simulink model "Target_Control_System"  (R2021b)
settings: Solver=FixedStepDiscrete  StartTime=0.0  StopTime=5  RelTol=1e-3
PreLoadFcn:
  | RTWConfigurationCB('preloadfcn', bdroot);
PostLoadFcn:
  | load('configuration/data_struct.mat');
  | load('configuration/fluxMaps_propMotor.mat');
  | load('configuration/parameterInit_PROP.mat');
  | load('configuration/parameterInit_PUMP.mat');
  | load('configuration/parameterInit_PITCH.mat');
  | load('configuration/parameterInit_TILT.mat');
  | %load('configuration/base_workspace_signal_definition.mat');
  | %load('resolvedatastores_to_baseworkspace_for_faster_simulation.mat');
model workspace (MAT data in the model file):
  SIMULATION_OPTIONS : Simulink.Parameter (value not decoded)
  TARGET_CODE_GEN : Simulink.Parameter (value not decoded)
  TCS_SAMPLE_FREQ_HZ : Simulink.Parameter (value not decoded)
symbols that are objects in the model workspace (value not decoded): TARGET_CODE_GEN, TCS_SAMPLE_FREQ_HZ
undefined symbols (not defined in the file): A_DQ_REF_LPF_INIT__PITCH, A_DQ_REF_LPF_INIT__PROP, A_DQ_REF_LPF_INIT__PUMP, A_DQ_REF_LPF_INIT__TILT, A_OBSERVER_CONFIDENCE_INIT__PITCH, A_OBSERVER_CONFIDENCE_INIT__PROP, A_OBSERVER_CONFIDENCE_INIT__PUMP, A_OBSERVER_CONFIDENCE_INIT__TILT, ACTUATOR_MAX_ANGLE_TRIP__PITCH, ACTUATOR_MIN_ANGLE_TRIP__PITCH, ACTUATOR_POS_SENSOR_INV_DIRECTION__PITCH, ACTUATOR_POS_SENSOR_INV_DIRECTION__TILT, ACTUATOR_POS_SENSOR_OFFSET__PITCH, ACTUATOR_POS_SENSOR_OFFSET__TILT, ADC_scaler1_baseaddr_TILT, ADC_SCALER_FLOAT_TO_FIXPOINT_EXPANSION, ANGLE_ELEC_FROM_SENSOR_OFFSET_INIT__PITCH, ANGLE_ELEC_FROM_SENSOR_OFFSET_INIT__PROP, ANGLE_ELEC_FROM_SENSOR_OFFSET_INIT__PUMP, ANGLE_ELEC_FROM_SENSOR_OFFSET_INIT__TILT, AUTO_CLEAR_FAULTS_ENABLED__PITCH, AUTO_CLEAR_FAULTS_ENABLED__PROP, AUTO_CLEAR_FAULTS_ENABLED__PUMP, AUTO_CLEAR_FAULTS_ENABLED__TILT, AUTO_CLEAR_FAULTS_WAIT_TICKS__PITCH, AUTO_CLEAR_FAULTS_WAIT_TICKS__PROP, AUTO_CLEAR_FAULTS_WAIT_TICKS__PUMP, AUTO_CLEAR_FAULTS_WAIT_TICKS__TILT, AUTO_I_ZERO_IDLE_TICKS__PITCH, AUTO_I_ZERO_IDLE_TICKS__PROP, AUTO_I_ZERO_IDLE_TICKS__PUMP, AUTO_I_ZERO_IDLE_TICKS__TILT, AUTO_I_ZERO_OFFSET_IDC_THRESHOLD__PITCH, AUTO_I_ZERO_OFFSET_IDC_THRESHOLD__PROP, AUTO_I_ZERO_OFFSET_IDC_THRESHOLD__PUMP, AUTO_I_ZERO_OFFSET_IDC_THRESHOLD__TILT, AUTO_I_ZERO_OFFSET_IPH_THRESHOLD__PITCH, AUTO_I_ZERO_OFFSET_IPH_THRESHOLD__PROP, AUTO_I_ZERO_OFFSET_IPH_THRESHOLD__PUMP, AUTO_I_ZERO_OFFSET_IPH_THRESHOLD__TILT, AUTO_SENSORLESS_SWITCHOVER_DISABLE_OMEGA, AUTO_SENSORLESS_SWITCHOVER_ENABLE_OMEGA, AUTO_SENSORLESS_SWITCHOVER_MIN_CONFIDENCE, AUXILIARY_PROTECTION_UNIT_BASEADDR__TILT, blanking_max_error_omega_INIT_PITCH, blanking_max_error_omega_INIT_TILT, blanking_max_error_position_INIT_PITCH, blanking_max_error_position_INIT_TILT, BRUTE_START_I_Q_REF_RAMP_SPEED__PITCH, BRUTE_START_I_Q_REF_RAMP_SPEED__PROP, BRUTE_START_I_Q_REF_RAMP_SPEED__PUMP, BRUTE_START_I_Q_REF_RAMP_SPEED__TILT, CONTROL_LOOP_DT_INIT__PITCH, CONTROL_LOOP_DT_INIT__PROP, CONTROL_LOOP_DT_INIT__PUMP, CONTROL_LOOP_DT_INIT__TILT, CORRECTION_FILTER_SCALE__PITCH, CORRECTION_FILTER_SCALE__PROP, CORRECTION_FILTER_SCALE__PUMP, CORRECTION_FILTER_SCALE__TILT ... (+458)
libraries: simulink x178, Reusables_Lib x24
(part 45 of 47)

== stateflow chart Target_Control_System/MainLoop/tiltMotor_mainLoop/mainTask_tilt/motorTaskMainFastStep(&oTilt)/Software Overcurrent Protection - Tilt/softwareOvercurrentProtection ==
  state Start
  state Drive_trip
    // Disable the drive and enter a trip state (error state)
    entry:
    oTilt.oMot_.oOut_.uiEnableGateDrive_ = 0;
    oTilt.oMot_.oOut_.uiCurrentControllerActive_ = 0;
    // NOTE: the actual turning off is done in the ctrl interrupt
    // formerly: Xil_Out32(uiGateDriverBaseaddr_, 0x0);
  state Store_previous_fault
    // If we were already in a fault state, store the previous fault:
    entry:
    oTilt.oMot_.oOut_.uiLastFaultState_ = oTilt.oMot_.oState_.uiDriveState_;
  state setTripState
    entry:
    oTilt.oMot_.oState_.uiDriveState_ = 1007;
  (default) -> Start
  Start -> (junction 7) : [oTilt.oMot_.oIn_.fIPhaseMagnitude_ > oTilt.oMot_.oParam_.fTripLimitSoftwareA_]
  (junction 7) -> Drive_trip [order 1] : [oTilt.oMot_.oState_.uiDriveState_ >= 200]
  (junction 7) -> (junction 10) [order 2]
  Drive_trip -> (junction 10)
  (junction 10) -> Store_previous_fault [order 1] : [oTilt.oMot_.oState_.uiDriveState_ >= 1000]
  (junction 10) -> setTripState [order 2]
  Store_previous_fault -> setTripState
  data: oTilt data_store_memory

== stateflow chart Target_Control_System/MainLoop/pitchMotor_mainLoop/Decimation gate for 200 Hz Pitch/Function-Call Subsystem/DClink_overCurrentProtection/Chart ==
  state Start
  state Drive_trip
    // Disable the drive and enter a trip state (error state)
    entry:
    oPitch.oMot_.oOut_.uiEnableGateDrive_ = 0;
    oPitch.oMot_.oOut_.uiCurrentControllerActive_ = 0;
    // NOTE: the actual turning off is done in the ctrl interrupt
    // formerly: Xil_Out32(uiGateDriverBaseaddr_, 0x0);
  state Store_previous_fault
    // If we were already in a fault state, store the previous fault:
    entry:
    oPitch.oMot_.oOut_.uiLastFaultState_ = oPitch.oMot_.oState_.uiDriveState_;
  state setTripState
    entry:
    oPitch.oMot_.oState_.uiDriveState_ = DClink_tripCode;
  (default) -> Start
  Start -> (junction 11) [order 2] : [(oPitch.oMot_.oOut_.fIdcLpf_ < oPitch.oMot_.oParam_.fIdcMinTrip_) && ...
      | (oPitch.oMot_.oState_.uiDriveState_ < 1000)]
      | {DClink_tripCode = 1006;}
  Start -> (junction 11) [order 1] : [(oPitch.oMot_.oOut_.fIdcLpf_ > oPitch.oMot_.oParam_.fIdcMaxTrip_) && ...
      | (oPitch.oMot_.oState_.uiDriveState_ < 1000)]
      | {DClink_tripCode = 1005;}
  setTripState -> Start
  (junction 11) -> Drive_trip [order 1] : [oPitch.oMot_.oState_.uiDriveState_ >= 200]
  (junction 11) -> (junction 2) [order 2]
  Drive_trip -> (junction 2)
  (junction 2) -> Store_previous_fault [order 1] : [oPitch.oMot_.oState_.uiDriveState_ >= 1000]
  (junction 2) -> setTripState [order 2]
  Store_previous_fault -> setTripState
  data: oPitch data_store_memory; DClink_tripCode local double

== stateflow chart Target_Control_System/MainLoop/pitchMotor_mainLoop/Decimation gate for 200 Hz Pitch/Function-Call Subsystem/Position control checks/NOT position control mode/Chart ==
  state Start
  state Blanking_mode_inactive
    // Never blank in state 200
    entry:
    oPitch.oMot_.oState_.iRpmBlankingActive_ = 0;
  state Blanking_mode_active
    entry:
    oPitch.oMot_.oState_.iRpmBlankingActive_ = 1;
  (default) -> Start
  Blanking_mode_inactive -> Start
  Start -> (junction 5)
  (junction 6) -> Start [order 2]
  Blanking_mode_active -> Start
  (junction 5) -> (junction 6) [order 2]
  (junction 5) -> Blanking_mode_inactive [order 1] : [oPitch.oMot_.oState_.uiDriveState_ == 200 || ...
      | oPitch.oMot_.oState_.fObserverConfidence_ > oPitch.oMot_.oParam_.fRpmBlankingUnblankConfidence_]
  (junction 6) -> Blanking_mode_active [order 1] : [oPitch.oMot_.oState_.fObserverConfidence_ < ...
      | oPitch.oMot_.oParam_.fRpmBlankingBlankConfidence_]
  data: oPitch data_store_memory

== stateflow chart Target_Control_System/MainLoop/pitchMotor_mainLoop/Decimation gate for 200 Hz Pitch/Function-Call Subsystem/Position control checks/Position control mode/Check AD2S1210/Enabled Subsystem/Chart ==
  state Start
  state Drive_trip
    // Disable the drive and enter a trip state (error state)
    entry:
    oPitch.oMot_.oOut_.uiEnableGateDrive_ = 0;
    oPitch.oMot_.oOut_.uiCurrentControllerActive_ = 0;
    // NOTE: the actual turning off is done in the ctrl interrupt
    // formerly: Xil_Out32(uiGateDriverBaseaddr_, 0x0);
  state Store_previous_fault
    // If we were already in a fault state, store the previous fault:
    entry:
    oPitch.oMot_.oOut_.uiLastFaultState_ = oPitch.oMot_.oState_.uiDriveState_;
  state setTripState
    entry:
    oPitch.oMot_.oState_.uiDriveState_ = 1026;
  (default) -> Start
  setTripState -> Start
  Start -> (junction 6) : [oPitch.oMot_.oState_.opInputResolverData_.uiControlReadback_ != DEFAULT_RESOLVER_CONTROL_WORD]
      | // Normally, the value is 97d = 0x61.
  (junction 6) -> Drive_trip [order 1] : [oPitch.oMot_.oState_.uiDriveState_ >= 200]
  (junction 6) -> (junction 7) [order 2]
  Drive_trip -> (junction 7)
  (junction 7) -> Store_previous_fault [order 1] : [oPitch.oMot_.oState_.uiDriveState_ >= 1000]
  (junction 7) -> setTripState [order 2]
  Store_previous_fault -> setTripState
  data: oPitch data_store_memory; DEFAULT_RESOLVER_CONTROL_WORD parameter double

== stateflow chart Target_Control_System/MainLoop/pitchMotor_mainLoop/Decimation gate for 200 Hz Pitch/Function-Call Subsystem/Position control checks/Position control mode/Check fighting controllers/Enabled Subsystem/Enabled Subsystem/Chart ==
  state Start
  state not_fighting
    entry:
    oPitch.oMot_.oState_.oPosSensor_.iFightingConsecutiveStepsCounter_ = 0;
  state fighting
    entry:
    oPitch.oMot_.oState_.oPosSensor_.iFightingConsecutiveStepsCounter_++;
  state Drive_trip
    // Disable the drive and enter a trip state (error state)
    entry:
    oPitch.oMot_.oOut_.uiEnableGateDrive_ = 0;
    oPitch.oMot_.oOut_.uiCurrentControllerActive_ = 0;
    // NOTE: the actual turning off is done in the ctrl interrupt
    // formerly: Xil_Out32(uiGateDriverBaseaddr_, 0x0);
  state Store_previous_fault
    // If we were already in a fault state, store the previous fault:
    entry:
    oPitch.oMot_.oOut_.uiLastFaultState_ = oPitch.oMot_.oState_.uiDriveState_;
  state setTripState
    entry:
    oPitch.oMot_.oState_.uiDriveState_ = 1029;
  (default) -> Start
  setTripState -> Start
  fighting -> Start [order 2]
  Start -> (junction 48)
  not_fighting -> Start
  (junction 48) -> not_fighting [order 2]
  (junction 48) -> fighting [order 1] : [(fabs(oPitch.oMot_.oState_.fIqRefBeforeRamp_) > oPitch.oMot_.oState_.oPosSensor_.fFightingCurrentMagnitude_) && ...
      | (fabs(oPitch.oMot_.oIn_.fIqSetpoint_) > oPitch.oMot_.oState_.oPosSensor_.fFightingCurrentMagnitude_) && ...
      | oPitch.oMot_.oState_.fIqRefBeforeRamp_ * oPitch.oMot_.oIn_.fIqSetpoint_ < 0.0F]
      | // detect opposing signs by multiplying. 2*3(=ok) > 0 and -2*-3(=ok) > 0, but -2*3(=bad) < 0
  fighting -> (junction 16) [order 1] : [oPitch.oMot_.oState_.oPosSensor_.iFightingConsecutiveStepsCounter_ > oPitch.oMot_.oState_.oPosSensor_.iFightingConsecutiveSteps_]
  (junction 16) -> Drive_trip [order 1] : [oPitch.oMot_.oState_.uiDriveState_ >= 200]
  (junction 16) -> (junction 17) [order 2]
  Drive_trip -> (junction 17)
  (junction 17) -> Store_previous_fault [order 1] : [oPitch.oMot_.oState_.uiDriveState_ >= 1000]
  (junction 17) -> setTripState [order 2]
  Store_previous_fault -> setTripState
  data: oPitch data_store_memory

== stateflow chart Target_Control_System/MainLoop/pitchMotor_mainLoop/Decimation gate for 200 Hz Pitch/Function-Call Subsystem/Position control checks/Position control mode/Check for position halted/Chart1 ==
  state Start
  state position_halted
    // State 202 = Position halted; ignore external setpoint.
    oPitch.oMot_.oState_.oRampDataPos_.fSetpoint_ = oPitch.oMot_.oState_.oPosSensor_.fPositionHaltedSetpoint_;
  (default) -> Start
  position_halted -> Start
  Start -> position_halted : [oPitch.oMot_.oState_.uiDriveState_ == 202]
  data: oPitch data_store_memory

== stateflow chart Target_Control_System/MainLoop/pitchMotor_mainLoop/Decimation gate for 200 Hz Pitch/Function-Call Subsystem/Position control checks/Position control mode/checkSensorLimits(&oPitch)/Check broken sensor/All other sensor types/Chart ==
  state Start
  state Drive_trip1
    // Disable the drive and enter a trip state (error state)
    entry:
    oPitch.oMot_.oOut_.uiEnableGateDrive_ = 0;
    oPitch.oMot_.oOut_.uiCurrentControllerActive_ = 0;
    // NOTE: the actual turning off is done in the ctrl interrupt
    // formerly: Xil_Out32(uiGateDriverBaseaddr_, 0x0);
  state Store_previous_fault1
    // If we were already in a fault state, store the previous fault:
    entry:
    oPitch.oMot_.oOut_.uiLastFaultState_ = oPitch.oMot_.oState_.uiDriveState_;
  state setTripState1
    // Dead sensor
    entry:
    oPitch.oMot_.oState_.uiDriveState_ = inSensorTripCode;
  (default) -> Start
  Start -> (junction 52) [order 2] : [!(mdl_pitch_uiInputSensorFlags & 0x4)]
      | // target bit is active low
      | {inSensorTripCode = 1033;}
      | // broken sensor
  Start -> (junction 52) [order 1] : [mdl_pitch_uiInputSensorFlags & 0x1]
      | {inSensorTripCode = 1026;}
      | // dead sensor (no communication with the sensor)
  (junction 52) -> Drive_trip1 [order 1] : [oPitch.oMot_.oState_.uiDriveState_ >= 200]
  (junction 52) -> (junction 43) [order 2]
  Drive_trip1 -> (junction 43)
  (junction 43) -> Store_previous_fault1 [order 1] : [oPitch.oMot_.oState_.uiDriveState_ >= 1000]
  (junction 43) -> setTripState1 [order 2]
  Store_previous_fault1 -> setTripState1
  data: oPitch data_store_memory; mdl_pitch_uiInputSensorFlags data_store_memory; inSensorTripCode local double

== stateflow chart Target_Control_System/MainLoop/pitchMotor_mainLoop/Decimation gate for 200 Hz Pitch/Function-Call Subsystem/Position control checks/Position control mode/checkSensorLimits(&oPitch)/Check broken sensor/Resolver/Chart ==
  state Start
  state Drive_trip
    // Disable the drive and enter a trip state (error state)
    entry:
    oPitch.oMot_.oOut_.uiEnableGateDrive_ = 0;
    oPitch.oMot_.oOut_.uiCurrentControllerActive_ = 0;
    // NOTE: the actual turning off is done in the ctrl interrupt
    // formerly: Xil_Out32(uiGateDriverBaseaddr_, 0x0);
  state Store_previous_fault
    // If we were already in a fault state, store the previous fault:
    entry:
    oPitch.oMot_.oOut_.uiLastFaultState_ = oPitch.oMot_.oState_.uiDriveState_;
  state setTripState1
    // Dead sensor
    entry:
    oPitch.oMot_.oState_.uiDriveState_ = 1033;
  (default) -> Start
  setTripState1 -> Start
  Start -> (junction 147) : [mdl_pitch_uiInputSensorFlags & 0xF]
      | // broken resolver sensor
  (junction 147) -> Drive_trip [order 1] : [oPitch.oMot_.oState_.uiDriveState_ >= 200]
  (junction 147) -> (junction 143) [order 2]
  Drive_trip -> (junction 143)
  (junction 143) -> Store_previous_fault [order 1] : [oPitch.oMot_.oState_.uiDriveState_ >= 1000]
  (junction 143) -> setTripState1 [order 2]
  Store_previous_fault -> setTripState1
  data: oPitch data_store_memory; mdl_pitch_uiInputSensorFlags data_store_memory

== stateflow chart Target_Control_System/MainLoop/pitchMotor_mainLoop/Decimation gate for 200 Hz Pitch/Function-Call Subsystem/Position control checks/Position control mode/checkSensorLimits(&oPitch)/Check delta input-output/Enabled Subsystem/Chart ==
  state Start
  state Drive_trip
    // Disable the drive and enter a trip state (error state)
    entry:
    oPitch.oMot_.oOut_.uiEnableGateDrive_ = 0;
    oPitch.oMot_.oOut_.uiCurrentControllerActive_ = 0;
    // NOTE: the actual turning off is done in the ctrl interrupt
    // formerly: Xil_Out32(uiGateDriverBaseaddr_, 0x0);
  state Store_previous_fault
    // If we were already in a fault state, store the previous fault:
    entry:
    oPitch.oMot_.oOut_.uiLastFaultState_ = oPitch.oMot_.oState_.uiDriveState_;
  state setTripState
    // Only if the output sensor isn't dead.
    entry:
    oPitch.oMot_.oState_.uiDriveState_ = 1032;
  (default) -> Start
  setTripState -> Start
  (junction 23) -> Start [order 2]
  Start -> (junction 23) : [!(mdl_pitch_uiOutputSensorFlags & 0x1)]
      | // only if the sensor isn't dead
  (junction 23) -> (junction 8) [order 1] : [fabs(oPitch.oMot_.oState_.oPosSensor_.oGbx_.fCurrentOutputAngle_ - oPitch.oMot_.oState_.oPosSensor_.fActuatorAngleFromSensor_) > ...
      | oPitch.oMot_.oState_.oPosSensor_.fInputToOutputSensorMaxDifference_]
  (junction 8) -> Drive_trip [order 1] : [oPitch.oMot_.oState_.uiDriveState_ >= 200]
  (junction 8) -> (junction 9) [order 2]
  Drive_trip -> (junction 9)
  (junction 9) -> Store_previous_fault [order 1] : [oPitch.oMot_.oState_.uiDriveState_ >= 1000]
  (junction 9) -> setTripState [order 2]
  Store_previous_fault -> setTripState
  data: oPitch data_store_memory; mdl_pitch_uiOutputSensorFlags data_store_memory

== stateflow chart Target_Control_System/MainLoop/pitchMotor_mainLoop/Decimation gate for 200 Hz Pitch/Function-Call Subsystem/Position control checks/Position control mode/checkSensorLimits(&oPitch)/Check for stuck sensor/Enabled Subsystem/Chart ==
  state Start
  state Drive_trip
    // Disable the drive and enter a trip state (error state)
    entry:
    oPitch.oMot_.oOut_.uiEnableGateDrive_ = 0;
    oPitch.oMot_.oOut_.uiCurrentControllerActive_ = 0;
    // NOTE: the actual turning off is done in the ctrl interrupt
    // formerly: Xil_Out32(uiGateDriverBaseaddr_, 0x0);
  state Store_previous_fault
    // If we were already in a fault state, store the previous fault:
    entry:
    oPitch.oMot_.oOut_.uiLastFaultState_ = oPitch.oMot_.oState_.uiDriveState_;
  state setTripState
    entry:
    oPitch.oMot_.oState_.uiDriveState_ = 1031;
  (default) -> Start
  setTripState -> Start
  Start -> (junction 8) : // More logic might be added
      | [oPitch.oMot_.oOut_.fIqLpf_ > oPitch.oMot_.oState_.oPosSensor_.fStuckSensorFractionOfFullCurrent_ * oPitch.oMot_.oParam_.fISetpointMax_]
  (junction 8) -> Drive_trip [order 1] : [oPitch.oMot_.oState_.uiDriveState_ >= 200]
  (junction 8) -> (junction 9) [order 2]
  Drive_trip -> (junction 9)
  (junction 9) -> Store_previous_fault [order 1] : [oPitch.oMot_.oState_.uiDriveState_ >= 1000]
  (junction 9) -> setTripState [order 2]
  Store_previous_fault -> setTripState
  data: oPitch data_store_memory

== stateflow chart Target_Control_System/MainLoop/pitchMotor_mainLoop/Decimation gate for 200 Hz Pitch/Function-Call Subsystem/Position control checks/Position control mode/checkSensorLimits(&oPitch)/Check limits/Chart ==
  state Check_output_sensor_limits [parallel]
    settings: executionOrder=1
    state Start
    state Drive_trip
      // Disable the drive and enter a trip state (error state)
      entry:
      oPitch.oMot_.oOut_.uiEnableGateDrive_ = 0;
      oPitch.oMot_.oOut_.uiCurrentControllerActive_ = 0;
      // NOTE: the actual turning off is done in the ctrl interrupt
      // formerly: Xil_Out32(uiGateDriverBaseaddr_, 0x0);
    state Store_previous_fault
      // If we were already in a fault state, store the previous fault:
      entry:
      oPitch.oMot_.oOut_.uiLastFaultState_ = oPitch.oMot_.oState_.uiDriveState_;
    state setTripState
      // Output sensor too high (only if the sensor is not dead)
      entry:
      oPitch.oMot_.oState_.uiDriveState_ = outSensorFaultCode;
    (default) -> Check_output_sensor_limits.Start
    (junction 46) -> Check_output_sensor_limits.Start [order 3]
    Check_output_sensor_limits.Start -> (junction 46) : [!(mdl_pitch_uiOutputSensorFlags & 0x1)]
        | // only if sensor is not dead
    Check_output_sensor_limits.setTripState -> Check_output_sensor_limits.Start
    (junction 46) -> (junction 70) [order 1] : [oPitch.oMot_.oState_.oPosSensor_.fActuatorAngleFromSensor_ > ...
        | oPitch.oMot_.oState_.oPosSensor_.fActuatorSensorAngleMaxTrip_]
        | {outSensorFaultCode = 1022;}
    (junction 70) -> Check_output_sensor_limits.Drive_trip [order 1] : [oPitch.oMot_.oState_.uiDriveState_ >= 200]
    (junction 46) -> (junction 70) [order 2] : [oPitch.oMot_.oState_.oPosSensor_.fActuatorAngleFromSensor_ < ...
        | oPitch.oMot_.oState_.oPosSensor_.fActuatorSensorAngleMinTrip_]
        | {outSensorFaultCode = 1023;}
    (junction 70) -> (junction 15) [order 2]
    Check_output_sensor_limits.Drive_trip -> (junction 15)
    (junction 15) -> Check_output_sensor_limits.Store_previous_fault [order 1] : [oPitch.oMot_.oState_.uiDriveState_ >= 1000]
    (junction 15) -> Check_output_sensor_limits.setTripState [order 2]
    Check_output_sensor_limits.Store_previous_fault -> Check_output_sensor_limits.setTripState
  state Check_input_sensor_limits [parallel]
    settings: executionOrder=2
    state Start
    state Drive_trip
      // Disable the drive and enter a trip state (error state)
      entry:
      oPitch.oMot_.oOut_.uiEnableGateDrive_ = 0;
      oPitch.oMot_.oOut_.uiCurrentControllerActive_ = 0;
      // NOTE: the actual turning off is done in the ctrl interrupt
      // formerly: Xil_Out32(uiGateDriverBaseaddr_, 0x0);
    state Store_previous_fault
      // If we were already in a fault state, store the previous fault:
      entry:
      oPitch.oMot_.oOut_.uiLastFaultState_ = oPitch.oMot_.oState_.uiDriveState_;
    state setTripState
      // Output sensor too high (only if the sensor is not dead)
      entry:
      oPitch.oMot_.oState_.uiDriveState_ = inSensorFaultCode;
    (default) -> Check_input_sensor_limits.Start
    Check_input_sensor_limits.Start -> (junction 90) [order 2] : [oPitch.oMot_.oState_.oPosSensor_.oGbx_.fCurrentOutputAngle_ < ...
        | oPitch.oMot_.oState_.oPosSensor_.fGbxAngleMinTrip_]
        | {outSensorFaultCode = 1025;}
    Check_input_sensor_limits.Start -> (junction 90) [order 1] : [oPitch.oMot_.oState_.oPosSensor_.oGbx_.fCurrentOutputAngle_ > ...
        | oPitch.oMot_.oState_.oPosSensor_.fGbxAngleMaxTrip_]
        | {inSensorFaultCode = 1024;}
    Check_input_sensor_limits.setTripState -> Check_input_sensor_limits.Start
    (junction 90) -> Check_input_sensor_limits.Drive_trip [order 1] : [oPitch.oMot_.oState_.uiDriveState_ >= 200]
    (junction 90) -> (junction 82) [order 2]
    Check_input_sensor_limits.Drive_trip -> (junction 82)
    (junction 82) -> Check_input_sensor_limits.Store_previous_fault [order 1] : [oPitch.oMot_.oState_.uiDriveState_ >= 1000]
    (junction 82) -> Check_input_sensor_limits.setTripState [order 2]
    Check_input_sensor_limits.Store_previous_fault -> Check_input_sensor_limits.setTripState
  data: oPitch data_store_memory; outSensorFaultCode local double; inSensorFaultCode local double; mdl_pitch_uiOutputSensorFlags data_store_memory

== stateflow chart Target_Control_System/MainLoop/tiltMotor_mainLoop/Decimation gate for 200 Hz Tilt/motorTaskMainDecimationAStep(&oTilt)/Current offset nulling/initiateOffsetNulling(&oTilt)/Chart ==
  state Start
  state initiateOffsetNulling
    //We can only do this if idle
    entry:
    oTilt.oIsr_.oState_.fOffsetIntegratorIa_ = 0.0;
    oTilt.oIsr_.oState_.fOffsetIntegratorIb_ = 0.0;
    oTilt.oIsr_.oState_.fOffsetIntegratorIc_ = 0.0;
    oTilt.oIsr_.oState_.fOffsetIntegratorIdc_ = 0.0;
    oTilt.oMot_.oState_.uiDriveState_ = 95;
  (default) -> Start
  initiateOffsetNulling -> Start : [oTilt.oMot_.oState_.uiCurrentOffsetNullingPerformed_ == 1]
  Start -> initiateOffsetNulling : [oTilt.oMot_.oState_.uiDriveState_ >= 99 && ...
      | oTilt.oMot_.oState_.uiDriveState_ < 102]
  data: oTilt data_store_memory

== stateflow chart Target_Control_System/MainLoop/tiltMotor_mainLoop/Decimation gate for 200 Hz Tilt/motorTaskMainDecimationAStep(&oTilt)/DClink_overCurrentProtection/Chart ==
  state Start
  state Drive_trip
    // Disable the drive and enter a trip state (error state)
    entry:
    oTilt.oMot_.oOut_.uiEnableGateDrive_ = 0;
    oTilt.oMot_.oOut_.uiCurrentControllerActive_ = 0;
    // NOTE: the actual turning off is done in the ctrl interrupt
    // formerly: Xil_Out32(uiGateDriverBaseaddr_, 0x0);
  state Store_previous_fault
    // If we were already in a fault state, store the previous fault:
    entry:
    oTilt.oMot_.oOut_.uiLastFaultState_ = oTilt.oMot_.oState_.uiDriveState_;
  state setTripState
    entry:
    oTilt.oMot_.oState_.uiDriveState_ = DClink_tripCode;
  (default) -> Start
  Start -> (junction 11) [order 2] : [(oTilt.oMot_.oOut_.fIdcLpf_ < oTilt.oMot_.oParam_.fIdcMinTrip_) && ...
      | (oTilt.oMot_.oState_.uiDriveState_ < 1000)]
      | {DClink_tripCode = 1006;}
  Start -> (junction 11) [order 1] : [(oTilt.oMot_.oOut_.fIdcLpf_ > oTilt.oMot_.oParam_.fIdcMaxTrip_) && ...
      | (oTilt.oMot_.oState_.uiDriveState_ < 1000)]
      | {DClink_tripCode = 1005;}
  setTripState -> Start
  (junction 11) -> Drive_trip [order 1] : [oTilt.oMot_.oState_.uiDriveState_ >= 200]
  (junction 11) -> (junction 2) [order 2]
  Drive_trip -> (junction 2)
  (junction 2) -> Store_previous_fault [order 1] : [oTilt.oMot_.oState_.uiDriveState_ >= 1000]
  (junction 2) -> setTripState [order 2]
  Store_previous_fault -> setTripState
  data: oTilt data_store_memory; DClink_tripCode local double

== stateflow chart Target_Control_System/MainLoop/tiltMotor_mainLoop/Decimation gate for 200 Hz Tilt/motorTaskMainDecimationAStep(&oTilt)/Position control checks/NOT position control mode/Chart ==
  state Start
  state Blanking_mode_inactive
    // Never blank in state 200
    entry:
    oTilt.oMot_.oState_.iRpmBlankingActive_ = 0;
  state Blanking_mode_active
    entry:
    oTilt.oMot_.oState_.iRpmBlankingActive_ = 1;
  (default) -> Start
  Blanking_mode_inactive -> Start
  Start -> (junction 5)
  (junction 6) -> Start [order 2]
  Blanking_mode_active -> Start
  (junction 5) -> (junction 6) [order 2]
  (junction 5) -> Blanking_mode_inactive [order 1] : [oTilt.oMot_.oState_.uiDriveState_ == 200 || ...
      | oTilt.oMot_.oState_.fObserverConfidence_ > oTilt.oMot_.oParam_.fRpmBlankingUnblankConfidence_]
  (junction 6) -> Blanking_mode_active [order 1] : [oTilt.oMot_.oState_.fObserverConfidence_ < ...
      | oTilt.oMot_.oParam_.fRpmBlankingBlankConfidence_]
  data: oTilt data_store_memory

== stateflow chart Target_Control_System/MainLoop/tiltMotor_mainLoop/Decimation gate for 200 Hz Tilt/motorTaskMainDecimationAStep(&oTilt)/Position control checks/Position control mode/Check AD2S1210/Enabled Subsystem/Chart ==
  state Start
  state Drive_trip
    // Disable the drive and enter a trip state (error state)
    entry:
    oTilt.oMot_.oOut_.uiEnableGateDrive_ = 0;
    oTilt.oMot_.oOut_.uiCurrentControllerActive_ = 0;
    // NOTE: the actual turning off is done in the ctrl interrupt
    // formerly: Xil_Out32(uiGateDriverBaseaddr_, 0x0);
  state Store_previous_fault
    // If we were already in a fault state, store the previous fault:
    entry:
    oTilt.oMot_.oOut_.uiLastFaultState_ = oTilt.oMot_.oState_.uiDriveState_;
  state setTripState
    entry:
    oTilt.oMot_.oState_.uiDriveState_ = 1026;
  (default) -> Start
  setTripState -> Start
  Start -> (junction 6) : [oTilt.oMot_.oState_.opInputResolverData_.uiControlReadback_ != DEFAULT_RESOLVER_CONTROL_WORD]
      | // Normally, the value is 97d = 0x61.
  (junction 6) -> Drive_trip [order 1] : [oTilt.oMot_.oState_.uiDriveState_ >= 200]
  (junction 6) -> (junction 7) [order 2]
  Drive_trip -> (junction 7)
  (junction 7) -> Store_previous_fault [order 1] : [oTilt.oMot_.oState_.uiDriveState_ >= 1000]
  (junction 7) -> setTripState [order 2]
  Store_previous_fault -> setTripState
  data: oTilt data_store_memory; DEFAULT_RESOLVER_CONTROL_WORD parameter double

== stateflow chart Target_Control_System/MainLoop/tiltMotor_mainLoop/Decimation gate for 200 Hz Tilt/motorTaskMainDecimationAStep(&oTilt)/Position control checks/Position control mode/Check fighting controllers/Enabled Subsystem/Enabled Subsystem/Chart ==
  state Start
  state not_fighting
    entry:
    oTilt.oMot_.oState_.oPosSensor_.iFightingConsecutiveStepsCounter_ = 0;
  state fighting
    entry:
    oTilt.oMot_.oState_.oPosSensor_.iFightingConsecutiveStepsCounter_++;
  state Drive_trip
    // Disable the drive and enter a trip state (error state)
    entry:
    oTilt.oMot_.oOut_.uiEnableGateDrive_ = 0;
    oTilt.oMot_.oOut_.uiCurrentControllerActive_ = 0;
    // NOTE: the actual turning off is done in the ctrl interrupt
    // formerly: Xil_Out32(uiGateDriverBaseaddr_, 0x0);
  state Store_previous_fault
    // If we were already in a fault state, store the previous fault:
    entry:
    oTilt.oMot_.oOut_.uiLastFaultState_ = oTilt.oMot_.oState_.uiDriveState_;
  state setTripState
    entry:
    oTilt.oMot_.oState_.uiDriveState_ = 1029;
  (default) -> Start
  setTripState -> Start
  fighting -> Start [order 2]
  Start -> (junction 48)
  not_fighting -> Start
  (junction 48) -> not_fighting [order 2]
  (junction 48) -> fighting [order 1] : [(fabs(oTilt.oMot_.oState_.fIqRefBeforeRamp_) > oTilt.oMot_.oState_.oPosSensor_.fFightingCurrentMagnitude_) && ...
      | (fabs(oTilt.oMot_.oIn_.fIqSetpoint_) > oTilt.oMot_.oState_.oPosSensor_.fFightingCurrentMagnitude_) && ...
      | oTilt.oMot_.oState_.fIqRefBeforeRamp_ * oTilt.oMot_.oIn_.fIqSetpoint_ < 0.0F]
      | // detect opposing signs by multiplying. 2*3(=ok) > 0 and -2*-3(=ok) > 0, but -2*3(=bad) < 0
  fighting -> (junction 16) [order 1] : [oTilt.oMot_.oState_.oPosSensor_.iFightingConsecutiveStepsCounter_ > oTilt.oMot_.oState_.oPosSensor_.iFightingConsecutiveSteps_]
  (junction 16) -> Drive_trip [order 1] : [oTilt.oMot_.oState_.uiDriveState_ >= 200]
  (junction 16) -> (junction 17) [order 2]
  Drive_trip -> (junction 17)
  (junction 17) -> Store_previous_fault [order 1] : [oTilt.oMot_.oState_.uiDriveState_ >= 1000]
  (junction 17) -> setTripState [order 2]
  Store_previous_fault -> setTripState
  data: oTilt data_store_memory

== stateflow chart Target_Control_System/MainLoop/tiltMotor_mainLoop/Decimation gate for 200 Hz Tilt/motorTaskMainDecimationAStep(&oTilt)/Position control checks/Position control mode/Check for position halted/Chart1 ==
  state Start
  state position_halted
    // State 202 = Position halted; ignore external setpoint.
    oTilt.oMot_.oState_.oRampDataPos_.fSetpoint_ = oTilt.oMot_.oState_.oPosSensor_.fPositionHaltedSetpoint_;
  (default) -> Start
  position_halted -> Start
  Start -> position_halted : [oTilt.oMot_.oState_.uiDriveState_ == 202]
  data: oTilt data_store_memory

== stateflow chart Target_Control_System/MainLoop/tiltMotor_mainLoop/Decimation gate for 200 Hz Tilt/motorTaskMainDecimationAStep(&oTilt)/Position control checks/Position control mode/checkSensorLimits(&oTilt)/Check broken sensor/All other sensor types/Chart ==
  state Start
  state Drive_trip1
    // Disable the drive and enter a trip state (error state)
    entry:
    oTilt.oMot_.oOut_.uiEnableGateDrive_ = 0;
    oTilt.oMot_.oOut_.uiCurrentControllerActive_ = 0;
    // NOTE: the actual turning off is done in the ctrl interrupt
    // formerly: Xil_Out32(uiGateDriverBaseaddr_, 0x0);
  state Store_previous_fault1
    // If we were already in a fault state, store the previous fault:
    entry:
    oTilt.oMot_.oOut_.uiLastFaultState_ = oTilt.oMot_.oState_.uiDriveState_;
  state setTripState
    // Dead sensor
    entry:
    oTilt.oMot_.oState_.uiDriveState_ = inSensorTripCode;
  (default) -> Start
  Start -> (junction 52) [order 2] : [!(mdl_tilt_uiInputSensorFlags & 0x4)]
      | // target bit is active low
      | {inSensorTripCode = 1033;}
      | // broken sensor
  Start -> (junction 52) [order 1] : [mdl_tilt_uiInputSensorFlags & 0x1]
      | {inSensorTripCode = 1026;}
      | // dead sensor (no communication with the sensor)
  (junction 52) -> Drive_trip1 [order 1] : [oTilt.oMot_.oState_.uiDriveState_ >= 200]
  (junction 52) -> (junction 43) [order 2]
  Drive_trip1 -> (junction 43)
  (junction 43) -> Store_previous_fault1 [order 1] : [oTilt.oMot_.oState_.uiDriveState_ >= 1000]
  (junction 43) -> setTripState [order 2]
  Store_previous_fault1 -> setTripState
  data: oTilt data_store_memory; mdl_tilt_uiInputSensorFlags data_store_memory; inSensorTripCode local double

== stateflow chart Target_Control_System/MainLoop/tiltMotor_mainLoop/Decimation gate for 200 Hz Tilt/motorTaskMainDecimationAStep(&oTilt)/Position control checks/Position control mode/checkSensorLimits(&oTilt)/Check broken sensor/Resolver/Chart ==
  state Start
  state Drive_trip
    // Disable the drive and enter a trip state (error state)
    entry:
    oTilt.oMot_.oOut_.uiEnableGateDrive_ = 0;
    oTilt.oMot_.oOut_.uiCurrentControllerActive_ = 0;
    // NOTE: the actual turning off is done in the ctrl interrupt
    // formerly: Xil_Out32(uiGateDriverBaseaddr_, 0x0);
  state Store_previous_fault
    // If we were already in a fault state, store the previous fault:
    entry:
    oTilt.oMot_.oOut_.uiLastFaultState_ = oTilt.oMot_.oState_.uiDriveState_;
  state setTripState
    // Dead sensor
    entry:
    oTilt.oMot_.oState_.uiDriveState_ = 1033;
  (default) -> Start
  setTripState -> Start
  Start -> (junction 147) : [mdl_tilt_uiInputSensorFlags & 0xF]
      | // broken resolver sensor
  (junction 147) -> Drive_trip [order 1] : [oTilt.oMot_.oState_.uiDriveState_ >= 200]
  (junction 147) -> (junction 143) [order 2]
  Drive_trip -> (junction 143)
  (junction 143) -> Store_previous_fault [order 1] : [oTilt.oMot_.oState_.uiDriveState_ >= 1000]
  (junction 143) -> setTripState [order 2]
  Store_previous_fault -> setTripState
  data: oTilt data_store_memory; mdl_tilt_uiInputSensorFlags data_store_memory

== stateflow chart Target_Control_System/MainLoop/tiltMotor_mainLoop/Decimation gate for 200 Hz Tilt/motorTaskMainDecimationAStep(&oTilt)/Position control checks/Position control mode/checkSensorLimits(&oTilt)/Check delta input-output/Enabled Subsystem/Chart ==
  state Start
  state Drive_trip
    // Disable the drive and enter a trip state (error state)
    entry:
    oTilt.oMot_.oOut_.uiEnableGateDrive_ = 0;
    oTilt.oMot_.oOut_.uiCurrentControllerActive_ = 0;
    // NOTE: the actual turning off is done in the ctrl interrupt
    // formerly: Xil_Out32(uiGateDriverBaseaddr_, 0x0);
  state Store_previous_fault
    // If we were already in a fault state, store the previous fault:
    entry:
    oTilt.oMot_.oOut_.uiLastFaultState_ = oTilt.oMot_.oState_.uiDriveState_;
  state setTripState
    // Only if the output sensor isn't dead.
    entry:
    oTilt.oMot_.oState_.uiDriveState_ = 1032;
  (default) -> Start
  setTripState -> Start
  (junction 23) -> Start [order 2]
  Start -> (junction 23) : [!(mdl_tilt_uiOutputSensorFlags & 0x1)]
      | // only if the sensor isn't dead
  (junction 23) -> (junction 8) [order 1] : [fabs(oTilt.oMot_.oState_.oPosSensor_.oGbx_.fCurrentOutputAngle_ - oTilt.oMot_.oState_.oPosSensor_.fActuatorAngleFromSensor_) > ...
      | oTilt.oMot_.oState_.oPosSensor_.fInputToOutputSensorMaxDifference_]
  (junction 8) -> Drive_trip [order 1] : [oTilt.oMot_.oState_.uiDriveState_ >= 200]
  (junction 8) -> (junction 9) [order 2]
  Drive_trip -> (junction 9)
  (junction 9) -> Store_previous_fault [order 1] : [oTilt.oMot_.oState_.uiDriveState_ >= 1000]
  (junction 9) -> setTripState [order 2]
  Store_previous_fault -> setTripState
  data: oTilt data_store_memory; mdl_tilt_uiOutputSensorFlags data_store_memory

== stateflow chart Target_Control_System/MainLoop/tiltMotor_mainLoop/Decimation gate for 200 Hz Tilt/motorTaskMainDecimationAStep(&oTilt)/Position control checks/Position control mode/checkSensorLimits(&oTilt)/Check for stuck sensor/Enabled Subsystem/Chart ==
  state Start
  state Drive_trip
    // Disable the drive and enter a trip state (error state)
    entry:
    oTilt.oMot_.oOut_.uiEnableGateDrive_ = 0;
    oTilt.oMot_.oOut_.uiCurrentControllerActive_ = 0;
    // NOTE: the actual turning off is done in the ctrl interrupt
    // formerly: Xil_Out32(uiGateDriverBaseaddr_, 0x0);
  state Store_previous_fault
    // If we were already in a fault state, store the previous fault:
    entry:
    oTilt.oMot_.oOut_.uiLastFaultState_ = oTilt.oMot_.oState_.uiDriveState_;
  state setTripState
    entry:
    oTilt.oMot_.oState_.uiDriveState_ = 1031;
  (default) -> Start
  setTripState -> Start
  Start -> (junction 8) : // More logic might be added
      | [oTilt.oMot_.oOut_.fIqLpf_ > oTilt.oMot_.oState_.oPosSensor_.fStuckSensorFractionOfFullCurrent_ * oTilt.oMot_.oParam_.fISetpointMax_]
  (junction 8) -> Drive_trip [order 1] : [oTilt.oMot_.oState_.uiDriveState_ >= 200]
  (junction 8) -> (junction 9) [order 2]
  Drive_trip -> (junction 9)
  (junction 9) -> Store_previous_fault [order 1] : [oTilt.oMot_.oState_.uiDriveState_ >= 1000]
  (junction 9) -> setTripState [order 2]
  Store_previous_fault -> setTripState
  data: oTilt data_store_memory

== stateflow chart Target_Control_System/MainLoop/tiltMotor_mainLoop/Decimation gate for 200 Hz Tilt/motorTaskMainDecimationAStep(&oTilt)/Position control checks/Position control mode/checkSensorLimits(&oTilt)/Check limits/Chart ==
  state Check_output_sensor_limits [parallel]
    settings: executionOrder=1
    state Start
    state Drive_trip
      // Disable the drive and enter a trip state (error state)
      entry:
      oTilt.oMot_.oOut_.uiEnableGateDrive_ = 0;
      oTilt.oMot_.oOut_.uiCurrentControllerActive_ = 0;
      // NOTE: the actual turning off is done in the ctrl interrupt
      // formerly: Xil_Out32(uiGateDriverBaseaddr_, 0x0);
    state Store_previous_fault
      // If we were already in a fault state, store the previous fault:
      entry:
      oTilt.oMot_.oOut_.uiLastFaultState_ = oTilt.oMot_.oState_.uiDriveState_;
    state setTripState
      // Output sensor too high (only if the sensor is not dead)
      entry:
      oTilt.oMot_.oState_.uiDriveState_ = outSensorFaultCode;
    (default) -> Check_output_sensor_limits.Start
    (junction 46) -> Check_output_sensor_limits.Start [order 3]
    Check_output_sensor_limits.Start -> (junction 46) : [!(mdl_tilt_uiOutputSensorFlags & 0x1)]
        | // only if sensor is not dead
    Check_output_sensor_limits.setTripState -> Check_output_sensor_limits.Start
    (junction 46) -> (junction 70) [order 1] : [oTilt.oMot_.oState_.oPosSensor_.fActuatorAngleFromSensor_ > ...
        | oTilt.oMot_.oState_.oPosSensor_.fActuatorSensorAngleMaxTrip_]
        | {outSensorFaultCode = 1022;}
    (junction 70) -> Check_output_sensor_limits.Drive_trip [order 1] : [oTilt.oMot_.oState_.uiDriveState_ >= 200]
    (junction 46) -> (junction 70) [order 2] : [oTilt.oMot_.oState_.oPosSensor_.fActuatorAngleFromSensor_ < ...
        | oTilt.oMot_.oState_.oPosSensor_.fActuatorSensorAngleMinTrip_]
        | {outSensorFaultCode = 1023;}
    (junction 70) -> (junction 15) [order 2]
    Check_output_sensor_limits.Drive_trip -> (junction 15)
    (junction 15) -> Check_output_sensor_limits.Store_previous_fault [order 1] : [oTilt.oMot_.oState_.uiDriveState_ >= 1000]
    (junction 15) -> Check_output_sensor_limits.setTripState [order 2]
    Check_output_sensor_limits.Store_previous_fault -> Check_output_sensor_limits.setTripState
  state Check_input_sensor_limits [parallel]
    settings: executionOrder=2
    state Start
    state Drive_trip
      // Disable the drive and enter a trip state (error state)
      entry:
      oTilt.oMot_.oOut_.uiEnableGateDrive_ = 0;
      oTilt.oMot_.oOut_.uiCurrentControllerActive_ = 0;
      // NOTE: the actual turning off is done in the ctrl interrupt
      // formerly: Xil_Out32(uiGateDriverBaseaddr_, 0x0);
    state Store_previous_fault
      // If we were already in a fault state, store the previous fault:
      entry:
      oTilt.oMot_.oOut_.uiLastFaultState_ = oTilt.oMot_.oState_.uiDriveState_;
    state setTripState
      // Output sensor too high (only if the sensor is not dead)
      entry:
      oTilt.oMot_.oState_.uiDriveState_ = inSensorFaultCode;
    (default) -> Check_input_sensor_limits.Start
    Check_input_sensor_limits.Start -> (junction 90) [order 2] : [oTilt.oMot_.oState_.oPosSensor_.oGbx_.fCurrentOutputAngle_ < ...
        | oTilt.oMot_.oState_.oPosSensor_.fGbxAngleMinTrip_]
        | {outSensorFaultCode = 1025;}
    Check_input_sensor_limits.Start -> (junction 90) [order 1] : [oTilt.oMot_.oState_.oPosSensor_.oGbx_.fCurrentOutputAngle_ > ...
        | oTilt.oMot_.oState_.oPosSensor_.fGbxAngleMaxTrip_]
        | {inSensorFaultCode = 1024;}
    Check_input_sensor_limits.setTripState -> Check_input_sensor_limits.Start
    (junction 90) -> Check_input_sensor_limits.Drive_trip [order 1] : [oTilt.oMot_.oState_.uiDriveState_ >= 200]
    (junction 90) -> (junction 82) [order 2]
    Check_input_sensor_limits.Drive_trip -> (junction 82)
    (junction 82) -> Check_input_sensor_limits.Store_previous_fault [order 1] : [oTilt.oMot_.oState_.uiDriveState_ >= 1000]
    (junction 82) -> Check_input_sensor_limits.setTripState [order 2]
    Check_input_sensor_limits.Store_previous_fault -> Check_input_sensor_limits.setTripState
  data: oTilt data_store_memory; outSensorFaultCode local double; inSensorFaultCode local double; mdl_tilt_uiOutputSensorFlags data_store_memory

== stateflow chart Target_Control_System/InterruptFunction/pitchMotor_isrTask/isrStateMachine/ISR State Machine ==
  state SuperState
    state ISR_States [parallel]
      // Main drive not active, just idle or various auxiliary operating modes
      // Do specific things:
      settings: executionOrder=1
      state Start
      state initiateCurrentOffsetNulling
        during:
        //Run an I controller for each current channel to be zerod, that zeros the actual reading
        // Note: the address to write out to
        oPitch.oIsr_.oState_.fOffsetIntegratorIa_ += oPitch.oIsr_.oIn_.oAdcData_.fIa_;
        oPitch.oIsr_.oOut_.iOffsetIa_ -= cast((500.0F*oPitch.oIsr_.oIn_.oAdcData_.fIa_ + 0.01F*oPitch.oIsr_.oState_.fOffsetIntegratorIa_), int32);
        oPitch.oIsr_.oState_.fOffsetIntegratorIb_ += oPitch.oIsr_.oIn_.oAdcData_.fIb_;
        oPitch.oIsr_.oOut_.iOffsetIb_ -= cast((500.0F*oPitch.oIsr_.oIn_.oAdcData_.fIb_ + 0.01F*oPitch.oIsr_.oState_.fOffsetIntegratorIb_), int32);
        oPitch.oIsr_.oState_.fOffsetIntegratorIc_ += oPitch.oIsr_.oIn_.oAdcData_.fIc_;
        oPitch.oIsr_.oOut_.iOffsetIc_ -= cast((500.0F*oPitch.oIsr_.oIn_.oAdcData_.fIc_ + 0.01F*oPitch.oIsr_.oState_.fOffsetIntegratorIc_), int32);
        oPitch.oIsr_.oState_.fOffsetIntegratorIdc_ += oPitch.oIsr_.oIn_.oAdcData_.fIdc_;
        oPitch.oIsr_.oOut_.iOffsetIdc_ -= cast((500.0F*oPitch.oIsr_.oIn_.oAdcData_.fIdc_ + 0.01F*oPitch.oIsr_.oState_.fOffsetIntegratorIdc_), int32);
        oPitch.oIsr_.oOut_.iIBiasUpdated_ = 1;
      state CaptureAverageVoltage
        during:
        //At 50% duty, capture intended average phase voltage
        oPitch.oIsr_.oState_.fOffsetAvgUphase_ += 0.001F * (oPitch.oIsr_.oIn_.oAdcData_.fUdc_ * 0.5F - oPitch.oIsr_.oState_.fOffsetAvgUphase_);
      state initiateVoltageOffsetNulling
        during:
        // At 50% duty, zero the voltage to the average voltage
        fTemp = oPitch.oIsr_.oIn_.oAdcData_.fUa_ - oPitch.oIsr_.oState_.fOffsetAvgUphase_;
        oPitch.oIsr_.oState_.fOffsetIntegratorUa_ += fTemp;
        oPitch.oIsr_.oOut_.iOffsetUa_ -= cast((50.0F * fTemp + 0.02F * oPitch.oIsr_.oState_.fOffsetIntegratorUa_), int32);
        fTemp = oPitch.oIsr_.oIn_.oAdcData_.fUb_ - oPitch.oIsr_.oState_.fOffsetAvgUphase_;
        oPitch.oIsr_.oState_.fOffsetIntegratorUb_ += fTemp;
        oPitch.oIsr_.oOut_.iOffsetUb_ -= cast((50.0F * fTemp + 0.01F * oPitch.oIsr_.oState_.fOffsetIntegratorUb_), int32);
        fTemp = oPitch.oIsr_.oIn_.oAdcData_.fUc_ - oPitch.oIsr_.oState_.fOffsetAvgUphase_;
        oPitch.oIsr_.oState_.fOffsetIntegratorUc_ += fTemp;
        oPitch.oIsr_.oOut_.iOffsetUc_ -= cast((50.0F * fTemp + 0.005F * oPitch.oIsr_.oState_.fOffsetIntegratorUc_), int32);
        oPitch.oIsr_.oOut_.iUBiasUpdated_ = 1;
      (default) -> Start
      Start -> initiateCurrentOffsetNulling [order 1] : [oPitch.oIsr_.oIn_.uiDriveState_ == 95]
      initiateCurrentOffsetNulling -> Start : [!(oPitch.oIsr_.oIn_.uiDriveState_ == 95)]
      Start -> CaptureAverageVoltage [order 2] : [oPitch.oIsr_.oIn_.uiDriveState_ == 250 || oPitch.oIsr_.oIn_.uiDriveState_ == 245]
      CaptureAverageVoltage -> Start : [!(oPitch.oIsr_.oIn_.uiDriveState_ == 250 || oPitch.oIsr_.oIn_.uiDriveState_ == 245)]
      Start -> initiateVoltageOffsetNulling [order 3] : [oPitch.oIsr_.oIn_.uiDriveState_ == 251 || oPitch.oIsr_.oIn_.uiDriveState_ == 246]
      initiateVoltageOffsetNulling -> Start : [!(oPitch.oIsr_.oIn_.uiDriveState_ == 251 || oPitch.oIsr_.oIn_.uiDriveState_ == 246)]
  (default) -> SuperState
  data: oPitch data_store_memory; fTemp local single

== stateflow chart Target_Control_System/MainLoop/pitchMotor_mainLoop/mainTask_pitch/motorTaskMainFastStep()/initiateOffsetNulling(&oPitch) ==
  state MainLoopFunctions
    state initiateOffsetNulling [parallel]
      settings: executionOrder=2
      state Disabled
      state Initiate
        entry:
        //We can only do this if idle
        oPitch.oIsr_.oState_.fOffsetIntegratorIa_ = 0.0;
        oPitch.oIsr_.oState_.fOffsetIntegratorIb_ = 0.0;
        oPitch.oIsr_.oState_.fOffsetIntegratorIc_ = 0.0;
        oPitch.oIsr_.oState_.fOffsetIntegratorIdc_ = 0.0;
        oPitch.oMot_.oState_.uiDriveState_ = 95;
      (default) -> MainLoopFunctions.initiateOffsetNulling.Disabled
      MainLoopFunctions.initiateOffsetNulling.Disabled -> Initiate : [oPitch.oMot_.oIn_.uiCurrentOffsetNullingActive_ == 1 ....
          | && (oPitch.oMot_.oState_.uiDriveState_ >= 99 ....
          |  || oPitch.oMot_.oState_.uiDriveState_ < 102)]
      Initiate -> MainLoopFunctions.initiateOffsetNulling.Disabled : [(oPitch.oMot_.oIn_.uiCurrentOffsetNullingActive_ == 0)]
    state initiateVoltageOffsetNulling [parallel]
      settings: executionOrder=1
      state Disabled
      state initiate
        entry:
        // Must do this at 50 % duty
        // Set the offsets to zero:
        fTemp = 0.5F;
        // In the future, there may be reasons to zero the offsets at duties different than 50%.
        // Set the target duty here
        oPitch.oMot_.oState_.uiDriveState_ = 245;
        oPitch.oMot_.oOut_.uiPwmRequestFromMain_ = 1;
        oPitch.oMot_.oOut_.uiPwmDutyTicksFromMainA_ = cast((fTemp * oPitch.oMot_.oParam_.fPwmPeriodTicksMainloopFloat_), uint32);
        oPitch.oMot_.oOut_.uiPwmDutyTicksFromMainB_ = cast((fTemp * oPitch.oMot_.oParam_.fPwmPeriodTicksMainloopFloat_), uint32);
        oPitch.oMot_.oOut_.uiPwmDutyTicksFromMainC_ = cast((fTemp * oPitch.oMot_.oParam_.fPwmPeriodTicksMainloopFloat_), uint32);
        oPitch.oMot_.oOut_.uiEnableGateDrive_ = 0x7;
      (default) -> MainLoopFunctions.initiateVoltageOffsetNulling.Disabled
      MainLoopFunctions.initiateVoltageOffsetNulling.Disabled -> (junction 277) : [oPitch.oMot_.oIn_.uiVoltageOffsetNullingActive_ == 1]
      (junction 277) -> MainLoopFunctions.initiateVoltageOffsetNulling.Disabled [order 1] : [oPitch.oMot_.oState_.uiDriveState_ < 100 ...
          |  || oPitch.oMot_.oState_.uiDriveState_ > 101] ...
          | // Only start if fully idle
      initiate -> MainLoopFunctions.initiateVoltageOffsetNulling.Disabled : [(oPitch.oMot_.oIn_.uiVoltageOffsetNullingActive_ == 0)]
      (junction 277) -> initiate [order 2]
  (default) -> MainLoopFunctions
  data: oPitch data_store_memory; fTemp local single

== stateflow chart Target_Control_System/MainLoop/tiltMotor_mainLoop/mainTask_tilt/motorTaskMainFastStep(&oTilt)/initiateOffsetNulling(&oTilt) ==
  state MainLoopFunctions
    state initiateOffsetNulling [parallel]
      settings: executionOrder=2
      state Disabled
      state Initiate
        entry:
        //We can only do this if idle
        oTilt.oIsr_.oState_.fOffsetIntegratorIa_ = 0.0;
        oTilt.oIsr_.oState_.fOffsetIntegratorIb_ = 0.0;
        oTilt.oIsr_.oState_.fOffsetIntegratorIc_ = 0.0;
        oTilt.oIsr_.oState_.fOffsetIntegratorIdc_ = 0.0;
        oTilt.oMot_.oState_.uiDriveState_ = 95;
      (default) -> MainLoopFunctions.initiateOffsetNulling.Disabled
      MainLoopFunctions.initiateOffsetNulling.Disabled -> Initiate : [oTilt.oMot_.oIn_.uiCurrentOffsetNullingActive_ == 1 ....
          | && (oTilt.oMot_.oState_.uiDriveState_ >= 99 ....
          |  || oTilt.oMot_.oState_.uiDriveState_ < 102)]
      Initiate -> MainLoopFunctions.initiateOffsetNulling.Disabled : [(oTilt.oMot_.oIn_.uiCurrentOffsetNullingActive_ == 0)]
    state initiateVoltageOffsetNulling [parallel]
      settings: executionOrder=1
      state Disabled
      state initiate
        entry:
        // Must do this at 50 % duty
        // Set the offsets to zero:
        fTemp = 0.5F;
        // In the future, there may be reasons to zero the offsets at duties different than 50%.
        // Set the target duty here
        oTilt.oMot_.oState_.uiDriveState_ = 245;
        oTilt.oMot_.oOut_.uiPwmRequestFromMain_ = 1;
        oTilt.oMot_.oOut_.uiPwmDutyTicksFromMainA_ = cast((fTemp * oTilt.oMot_.oParam_.fPwmPeriodTicksMainloopFloat_), uint32);
        oTilt.oMot_.oOut_.uiPwmDutyTicksFromMainB_ = cast((fTemp * oTilt.oMot_.oParam_.fPwmPeriodTicksMainloopFloat_), uint32);
        oTilt.oMot_.oOut_.uiPwmDutyTicksFromMainC_ = cast((fTemp * oTilt.oMot_.oParam_.fPwmPeriodTicksMainloopFloat_), uint32);
        oTilt.oMot_.oOut_.uiEnableGateDrive_ = 0x7;
      (default) -> MainLoopFunctions.initiateVoltageOffsetNulling.Disabled
      MainLoopFunctions.initiateVoltageOffsetNulling.Disabled -> (junction 277) : [oTilt.oMot_.oIn_.uiVoltageOffsetNullingActive_ == 1]
      (junction 277) -> MainLoopFunctions.initiateVoltageOffsetNulling.Disabled [order 1] : [oTilt.oMot_.oState_.uiDriveState_ < 100 ...
          |  || oTilt.oMot_.oState_.uiDriveState_ > 101] ...
          | // Only start if fully idle
      initiate -> MainLoopFunctions.initiateVoltageOffsetNulling.Disabled : [(oTilt.oMot_.oIn_.uiVoltageOffsetNullingActive_ == 0)]
      (junction 277) -> initiate [order 2]
  (default) -> MainLoopFunctions
  data: oTilt data_store_memory; fTemp local single
